simulink model "waveformSimulink_blocchi"  (R2019b)
settings: Solver=VariableStepAuto  StartTime=0.0  StopTime=1  RelTol=1e-3
values from neighbouring files (symbols this model uses):
  SNR = i    [start.m]
undefined symbols (not defined in the file or in its folder): Limit
libraries: commchan3 x4, commdigbbndcpm2 x4, dspsigops x4, commrandsrc3 x4, commsink2 x4, serdesDatapath x1
settings Model: Creator=boing  LastModifiedBy=Mattia

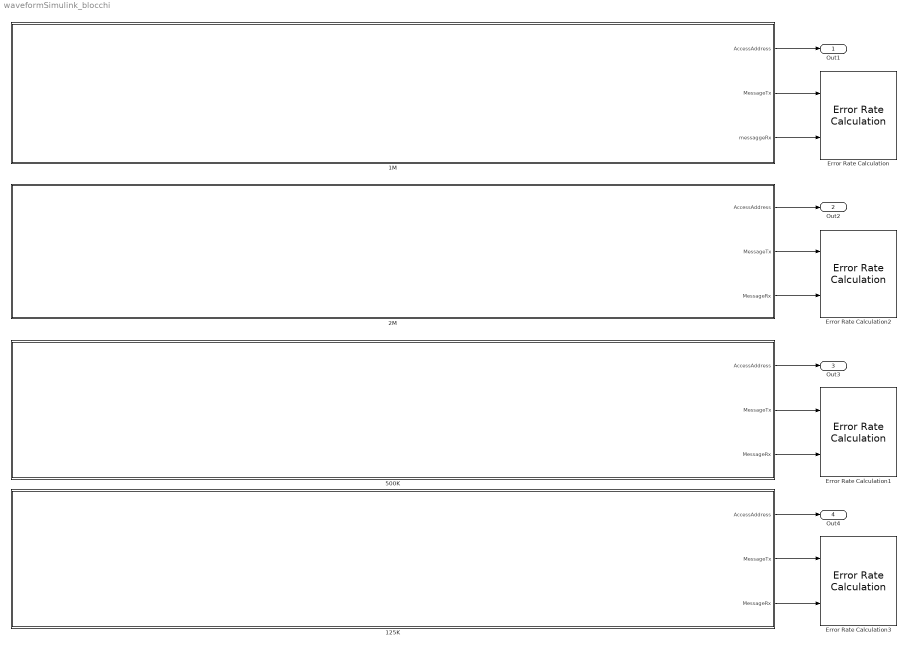
== system waveformSimulink_blocchi ==
  125K : Subsystem
  1M : Subsystem
  "2M " : Subsystem
  500K : Subsystem
  Error Rate Calculation : commsink2/Error Rate Calculation  N=0  st_delay=0  cp_mode=Entire frame  subframe=[]  PMode=Workspace  WsName=ErrorVec1M  RsMode2=off  stop=off  numErr=100  maxBits=1e6
      settings: SourceProductName=Communications Toolbox
  Error Rate Calculation1 : commsink2/Error Rate Calculation  N=0  st_delay=0  cp_mode=Entire frame  subframe=[]  PMode=Workspace  WsName=ErrorVec500K  RsMode2=off  stop=off  numErr=100  maxBits=1e6
      settings: SourceProductName=Communications Toolbox
  Error Rate Calculation2 : commsink2/Error Rate Calculation  N=0  st_delay=0  cp_mode=Entire frame  subframe=[]  PMode=Workspace  WsName=ErrorVec2M  RsMode2=off  stop=off  numErr=100  maxBits=1e6
      settings: SourceProductName=Communications Toolbox
  Error Rate Calculation3 : commsink2/Error Rate Calculation  N=0  st_delay=0  cp_mode=Entire frame  subframe=[]  PMode=Workspace  WsName=ErrorVec125K  RsMode2=off  stop=off  numErr=100  maxBits=1e6
      settings: SourceProductName=Communications Toolbox
  Out1 : Outport
  Out2 : Outport  Port=2
  Out3 : Outport  Port=3
  Out4 : Outport  Port=4
  wires:
  1M/2("MessageTx ") -> Error Rate Calculation/1
  1M/3(messaggeRx) -> Error Rate Calculation/2
  1M/1(AccessAddress) -> Out1/1
  500K/2(MessageTx) -> Error Rate Calculation1/1
  500K/3(MessageRx) -> Error Rate Calculation1/2
  "2M "/1(AccessAddress) -> Out2/1
  500K/1(AccessAddress) -> Out3/1
  "2M "/3(MessageRx) -> Error Rate Calculation2/2
  "2M "/2(MessageTx) -> Error Rate Calculation2/1
  125K/2(MessageTx) -> Error Rate Calculation3/1
  125K/3(MessageRx) -> Error Rate Calculation3/2
  125K/1(AccessAddress) -> Out4/1

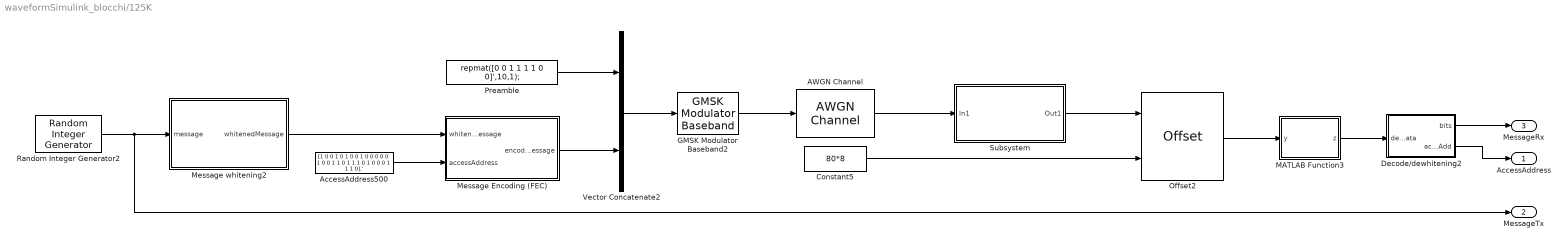
== system waveformSimulink_blocchi/125K ==
  AWGN Channel : commchan3/AWGN Channel  InputProcessing=Columns as channels (frame based)  seed=67  noiseMode="Signal to noise ratio  (SNR)"  EbNodB=10  EsNodB=10  SNRdB=SNR - 3  bitsPerSym=1  Ps=1  Tsym=1  variance=1
      settings: SourceProductName=Communications Toolbox
  AccessAddress500 : Constant  Value=[1 0 0 1 0 1 0 0 1 0 0 0 0 0 1 0 0 1 1 0 1 1 1 0 1 0 0 0 1 1 1 0].'  VectorParams1D=off
  Constant5 : Constant  Value=80*8
  Decode/dewhitening2 : MATLAB Function  TreatAsAtomicUnit=on
  GMSK Modulator Baseband2 : commdigbbndcpm2/GMSK Modulator Baseband  inputType=Bit  BT=0.5  pulseLength=1  preHistory=1  phaseOffset=4  samplesPerSymbol=8  RateOptions=Enforce single-rate processing  outDataType=double
      settings: SourceProductName=Communications Toolbox  SourceProductBaseCode=CM
  MATLAB Function3 : MATLAB Function  TreatAsAtomicUnit=on
  Message Encoding (FEC) : MATLAB Function  TreatAsAtomicUnit=on
  Message whitening2 : MATLAB Function  TreatAsAtomicUnit=on
  Offset2 : dspsigops/Offset  mode=Remove beginning samples  numDatOffPair=1  outWidthSpec=User-defined  outWidth=66560  actionOutRange=Clip
      settings: SourceProductName=DSP System Toolbox  SourceProductBaseCode=DS
  Preamble : Constant  Value=repmat([0 0 1 1 1 1 0 0]',10,1);
  Random Integer Generator2 : commrandsrc3/Random Integer Generator  SetSize=2  SeedSource=Auto  Seed=0  SampleTime=8*(10^-6)  SamplesPerFrame=1000  OutputDataType=double  SimulateUsing=Interpreted execution
      settings: SourceProductName=Communications Toolbox
  Subsystem : Subsystem
  Vector Concatenate2 : Concatenate
  AccessAddress : Outport
  MessageTx : Outport  Port=2
  MessageRx : Outport  Port=3
  wires:
  Vector Concatenate2/1 -> GMSK Modulator Baseband2/1
  Constant5/1 -> Offset2/2
  MATLAB Function3/1(z) -> Decode/dewhitening2/1(demodData)
  Decode/dewhitening2/1(bits) -> MessageRx/1
  Random Integer Generator2/1 -> MessageTx/1, Message whitening2/1(message)
  Offset2/1 -> MATLAB Function3/1(y)
  AccessAddress500/1 -> Message Encoding (FEC)/2(accessAddress)
  Decode/dewhitening2/2(accessAdd) -> AccessAddress/1
  Message Encoding (FEC)/1(encodedMessage) -> Vector Concatenate2/2
  Message whitening2/1(whitenedMessage) -> Message Encoding (FEC)/1(whitenedMessage)
  Preamble/1 -> Vector Concatenate2/1
  GMSK Modulator Baseband2/1 -> AWGN Channel/1
  AWGN Channel/1 -> Subsystem/1(In1)
  Subsystem/1(Out1) -> Offset2/1

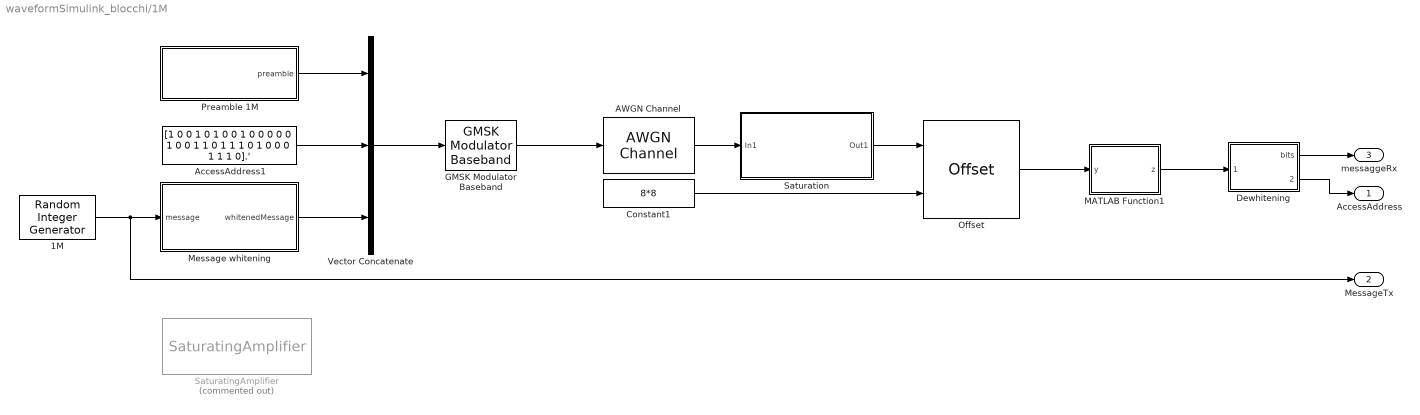
== system waveformSimulink_blocchi/1M ==
  1M : commrandsrc3/Random Integer Generator  SetSize=2  SeedSource=Auto  Seed=432234635  SampleTime=10^-6  SamplesPerFrame=1000  OutputDataType=double  SimulateUsing=Interpreted execution
      settings: SourceProductName=Communications Toolbox
  AWGN Channel : commchan3/AWGN Channel  InputProcessing=Columns as channels (frame based)  seed=67  noiseMode="Signal to noise ratio  (SNR)"  EbNodB=10  EsNodB=10  SNRdB=SNR  bitsPerSym=1  Ps=1  Tsym=1  variance=1
      settings: SourceProductName=Communications Toolbox
  "AccessAddress1 " : Constant  Value=[1 0 0 1 0 1 0 0 1 0 0 0 0 0 1 0 0 1 1 0 1 1 1 0 1 0 0 0 1 1 1 0].'  VectorParams1D=off
  Constant1 : Constant  Value=8*8
  Dewhitening : MATLAB Function  TreatAsAtomicUnit=on
  GMSK Modulator Baseband : commdigbbndcpm2/GMSK Modulator Baseband  inputType=Bit  BT=0.5  pulseLength=1  preHistory=1  phaseOffset=4  samplesPerSymbol=8  RateOptions=Enforce single-rate processing  outDataType=double
      settings: SourceProductName=Communications Toolbox  SourceProductBaseCode=CM
  MATLAB Function1 : MATLAB Function  TreatAsAtomicUnit=on
  Message whitening : MATLAB Function  TreatAsAtomicUnit=on
  Offset : dspsigops/Offset  mode=Remove beginning samples  numDatOffPair=1  outWidthSpec=User-defined  outWidth=8256  actionOutRange=Clip
      settings: SourceProductName=DSP System Toolbox  SourceProductBaseCode=DS
  Preamble 1M : MATLAB Function  TreatAsAtomicUnit=on
  SaturatingAmplifier : serdesDatapath/SaturatingAmplifier  Commented=on  InstantiateOnLoad=on  Mode=On  Specification=Limit and Linear Gain  Limit=1.2  LinearGain=1  VinVout=[ -2.4, -1.2; -1.92, -1.2; -1.44, -1.1328; -0.96, -0.86898; -0.48, -0.46862; 0, 0; 0.48, 0.46862; 0.96, 0.86898; 1.44, 1.1328; 1.92, 1.2; 2.4, 1.2 ]  ModeAMI=on  SavedName=SaturatingAmplifier
      settings: SourceProductName=SerDes Toolbox  SourceProductBaseCode=SX
  Saturation : Subsystem
  Vector Concatenate : Concatenate  NumInputs=3
  AccessAddress : Outport
  "MessageTx " : Outport  Port=2
  messaggeRx : Outport  Port=3
  wires:
  MATLAB Function1/1(z) -> Dewhitening/1(demodData)
  Message whitening/1(whitenedMessage) -> Vector Concatenate/3
  Offset/1 -> MATLAB Function1/1(y)
  Preamble 1M/1(preamble) -> Vector Concatenate/1
  Dewhitening/2(accessAdd) -> AccessAddress/1
  "AccessAddress1 "/1 -> Vector Concatenate/2
  Dewhitening/1(bits) -> messaggeRx/1
  Constant1/1 -> Offset/2
  Vector Concatenate/1 -> GMSK Modulator Baseband/1
  1M/1 -> "MessageTx "/1, Message whitening/1(message)
  GMSK Modulator Baseband/1 -> AWGN Channel/1
  AWGN Channel/1 -> Saturation/1(In1)
  Saturation/1(Out1) -> Offset/1

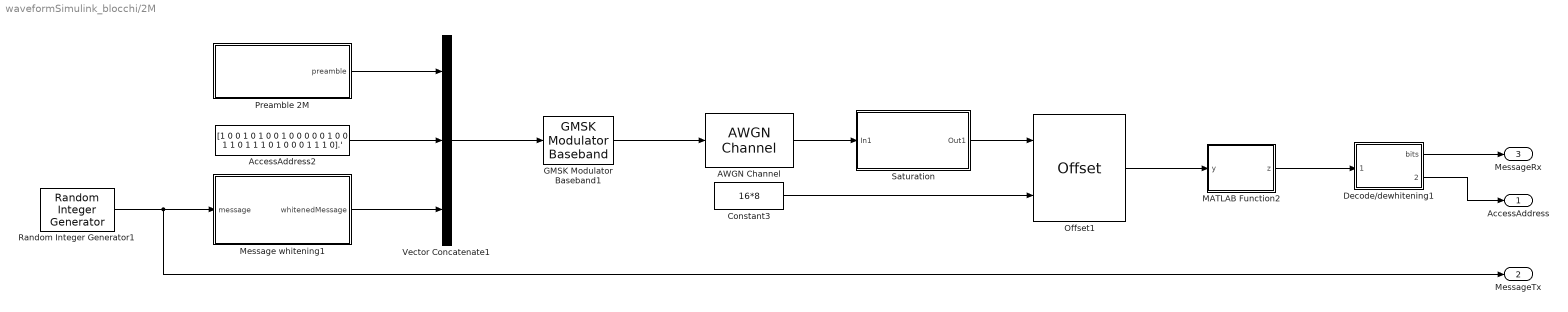
== system waveformSimulink_blocchi/2M  ==
  AWGN Channel : commchan3/AWGN Channel  InputProcessing=Columns as channels (frame based)  seed=67  noiseMode="Signal to noise ratio  (SNR)"  EbNodB=10  EsNodB=10  SNRdB=SNR  bitsPerSym=1  Ps=1  Tsym=1  variance=1
      settings: SourceProductName=Communications Toolbox
  AccessAddress2 : Constant  Value=[1 0 0 1 0 1 0 0 1 0 0 0 0 0 1 0 0 1 1 0 1 1 1 0 1 0 0 0 1 1 1 0].'  VectorParams1D=off
  Constant3 : Constant  Value=16*8
  Decode/dewhitening1 : MATLAB Function  TreatAsAtomicUnit=on
  GMSK Modulator Baseband1 : commdigbbndcpm2/GMSK Modulator Baseband  inputType=Bit  BT=0.5  pulseLength=1  preHistory=1  phaseOffset=4  samplesPerSymbol=8  RateOptions=Enforce single-rate processing  outDataType=double
      settings: SourceProductName=Communications Toolbox  SourceProductBaseCode=CM
  MATLAB Function2 : MATLAB Function  TreatAsAtomicUnit=on
  Message whitening1 : MATLAB Function  TreatAsAtomicUnit=on
  Offset1 : dspsigops/Offset  mode=Remove beginning samples  numDatOffPair=1  outWidthSpec=User-defined  outWidth=8256  actionOutRange=Clip
      settings: SourceProductName=DSP System Toolbox  SourceProductBaseCode=DS
  Preamble 2M : MATLAB Function  TreatAsAtomicUnit=on
  Random Integer Generator1 : commrandsrc3/Random Integer Generator  SetSize=2  SeedSource=Auto  Seed=0  SampleTime=0.5*(10^-6)  SamplesPerFrame=1000  OutputDataType=double  SimulateUsing=Interpreted execution
      settings: SourceProductName=Communications Toolbox
  "Saturation " : Subsystem
  Vector Concatenate1 : Concatenate  NumInputs=3
  AccessAddress : Outport
  MessageTx : Outport  Port=2
  MessageRx : Outport  Port=3
  wires:
  AccessAddress2/1 -> Vector Concatenate1/2
  Constant3/1 -> Offset1/2
  Preamble 2M/1(preamble) -> Vector Concatenate1/1
  Decode/dewhitening1/1(bits) -> MessageRx/1
  MATLAB Function2/1(z) -> Decode/dewhitening1/1(demodData)
  Vector Concatenate1/1 -> GMSK Modulator Baseband1/1
  Random Integer Generator1/1 -> MessageTx/1, Message whitening1/1(message)
  Decode/dewhitening1/2(accessAdd) -> AccessAddress/1
  Offset1/1 -> MATLAB Function2/1(y)
  Message whitening1/1(whitenedMessage) -> Vector Concatenate1/3
  GMSK Modulator Baseband1/1 -> AWGN Channel/1
  AWGN Channel/1 -> "Saturation "/1(In1)
  "Saturation "/1(Out1) -> Offset1/1

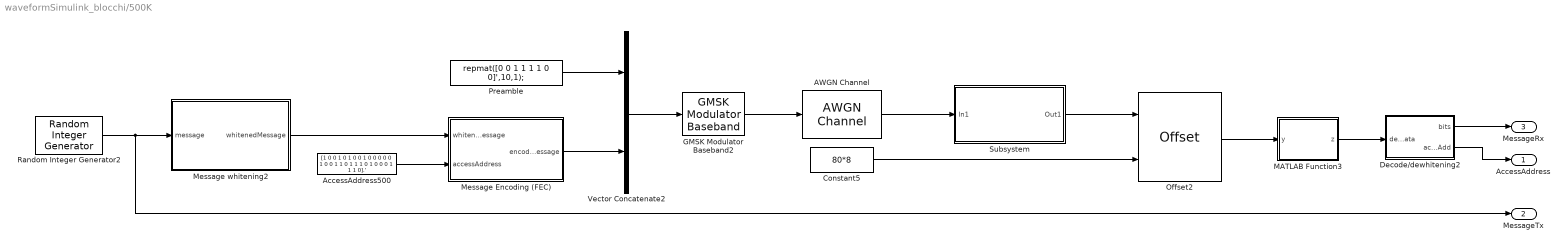
== system waveformSimulink_blocchi/500K ==
  AWGN Channel : commchan3/AWGN Channel  InputProcessing=Columns as channels (frame based)  seed=67  noiseMode="Signal to noise ratio  (SNR)"  EbNodB=10  EsNodB=10  SNRdB=SNR - 3  bitsPerSym=1  Ps=1  Tsym=1  variance=1
      settings: SourceProductName=Communications Toolbox
  AccessAddress500 : Constant  Value=[1 0 0 1 0 1 0 0 1 0 0 0 0 0 1 0 0 1 1 0 1 1 1 0 1 0 0 0 1 1 1 0].'  VectorParams1D=off
  Constant5 : Constant  Value=80*8
  Decode/dewhitening2 : MATLAB Function  TreatAsAtomicUnit=on
  GMSK Modulator Baseband2 : commdigbbndcpm2/GMSK Modulator Baseband  inputType=Bit  BT=0.5  pulseLength=1  preHistory=1  phaseOffset=4  samplesPerSymbol=8  RateOptions=Enforce single-rate processing  outDataType=double
      settings: SourceProductName=Communications Toolbox  SourceProductBaseCode=CM
  MATLAB Function3 : MATLAB Function  TreatAsAtomicUnit=on
  Message Encoding (FEC) : MATLAB Function  TreatAsAtomicUnit=on
  Message whitening2 : MATLAB Function  TreatAsAtomicUnit=on
  Offset2 : dspsigops/Offset  mode=Remove beginning samples  numDatOffPair=1  outWidthSpec=User-defined  outWidth=18416  actionOutRange=Clip
      settings: SourceProductName=DSP System Toolbox  SourceProductBaseCode=DS
  Preamble : Constant  Value=repmat([0 0 1 1 1 1 0 0]',10,1);
  Random Integer Generator2 : commrandsrc3/Random Integer Generator  SetSize=2  SeedSource=Auto  Seed=0  SampleTime=2*(10^-6)  SamplesPerFrame=1000  OutputDataType=double  SimulateUsing=Interpreted execution
      settings: SourceProductName=Communications Toolbox
  Subsystem : Subsystem
  Vector Concatenate2 : Concatenate
  AccessAddress : Outport
  MessageTx : Outport  Port=2
  MessageRx : Outport  Port=3
  wires:
  Vector Concatenate2/1 -> GMSK Modulator Baseband2/1
  Constant5/1 -> Offset2/2
  MATLAB Function3/1(z) -> Decode/dewhitening2/1(demodData)
  Decode/dewhitening2/1(bits) -> MessageRx/1
  Random Integer Generator2/1 -> MessageTx/1, Message whitening2/1(message)
  Offset2/1 -> MATLAB Function3/1(y)
  AccessAddress500/1 -> Message Encoding (FEC)/2(accessAddress)
  Decode/dewhitening2/2(accessAdd) -> AccessAddress/1
  Message Encoding (FEC)/1(encodedMessage) -> Vector Concatenate2/2
  Message whitening2/1(whitenedMessage) -> Message Encoding (FEC)/1(whitenedMessage)
  Preamble/1 -> Vector Concatenate2/1
  GMSK Modulator Baseband2/1 -> AWGN Channel/1
  AWGN Channel/1 -> Subsystem/1(In1)
  Subsystem/1(Out1) -> Offset2/1

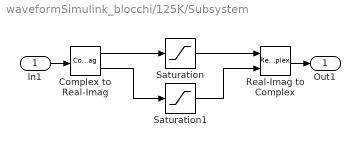
== system waveformSimulink_blocchi/125K/Subsystem ==
  In1 : Inport
  Complex to Real-Imag : ComplexToRealImag
  Real-Imag to Complex : RealImagToComplex
  Saturation : Saturate  UpperLimit=Limit  LowerLimit=-Limit
  Saturation1 : Saturate  UpperLimit=Limit  LowerLimit=-Limit
  Out1 : Outport
  wires:
  Complex to Real-Imag/1 -> Saturation/1
  Real-Imag to Complex/1 -> Out1/1
  Saturation/1 -> Real-Imag to Complex/1
  Saturation1/1 -> Real-Imag to Complex/2
  In1/1 -> Complex to Real-Imag/1
  Complex to Real-Imag/2 -> Saturation1/1

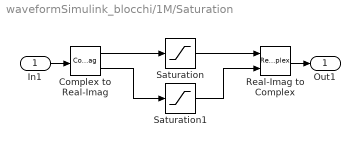
== system waveformSimulink_blocchi/1M/Saturation ==
  In1 : Inport
  Complex to Real-Imag : ComplexToRealImag
  Real-Imag to Complex : RealImagToComplex
  Saturation : Saturate  UpperLimit=Limit  LowerLimit=-Limit
  Saturation1 : Saturate  UpperLimit=Limit  LowerLimit=-Limit
  Out1 : Outport
  wires:
  Complex to Real-Imag/1 -> Saturation/1
  Real-Imag to Complex/1 -> Out1/1
  Saturation1/1 -> Real-Imag to Complex/2
  In1/1 -> Complex to Real-Imag/1
  Complex to Real-Imag/2 -> Saturation1/1
  Saturation/1 -> Real-Imag to Complex/1

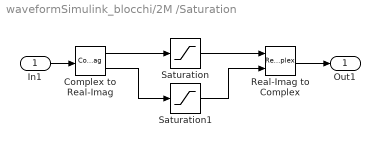
== system waveformSimulink_blocchi/2M /Saturation  ==
  In1 : Inport
  Complex to Real-Imag : ComplexToRealImag
  Real-Imag to Complex : RealImagToComplex
  Saturation : Saturate  UpperLimit=Limit  LowerLimit=-Limit
  Saturation1 : Saturate  UpperLimit=Limit  LowerLimit=-Limit
  Out1 : Outport
  wires:
  In1/1 -> Complex to Real-Imag/1
  Complex to Real-Imag/2 -> Saturation1/1
  Complex to Real-Imag/1 -> Saturation/1
  Saturation1/1 -> Real-Imag to Complex/2
  Real-Imag to Complex/1 -> Out1/1
  Saturation/1 -> Real-Imag to Complex/1

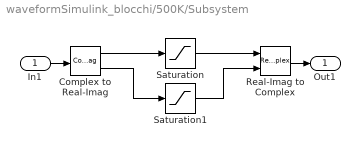
== system waveformSimulink_blocchi/500K/Subsystem ==
  In1 : Inport
  Complex to Real-Imag : ComplexToRealImag
  Real-Imag to Complex : RealImagToComplex
  Saturation : Saturate  UpperLimit=Limit  LowerLimit=-Limit
  Saturation1 : Saturate  UpperLimit=Limit  LowerLimit=-Limit
  Out1 : Outport
  wires:
  Complex to Real-Imag/2 -> Saturation1/1
  Complex to Real-Imag/1 -> Saturation/1
  Saturation1/1 -> Real-Imag to Complex/2
  Saturation/1 -> Real-Imag to Complex/1
  Real-Imag to Complex/1 -> Out1/1
  In1/1 -> Complex to Real-Imag/1

== matlab function waveformSimulink_blocchi/1M/Dewhitening ==
  data: demodData input; bits output double; accessAdd output
function [bits, accessAdd] = fcn(demodData)

accessAddLen = 32;      % Access address length in bits
chanIdx = 37;

% Demodulate and decodeaccessAdd
% if any(strcmp(phyMode,{'LE1M','LE2M'}))         % For LE1M or LE2M
accessAdd = int8(demodData(1:accessAddLen)>0);
decodeData = int8(demodData(1+accessAddLen:end)>0);
% else                                            % For LE500K or LE125K
%     [decodeData,accessAdd] = ble.internal.decode(demodData,phyMode);
% end

% Perform data dewhitening
dewhitenStateLen = 6;
chanIdxBin = comm.internal.utilities.de2biBase2LeftMSB(chanIdx,dewhitenStateLen);
initState = [1 chanIdxBin]; % Initial conditions of shift register
bits = double(ble.internal.whiten(decodeData,initState));

== matlab function waveformSimulink_blocchi/1M/Preamble 1M ==
  data: preamble output
function preamble = preamble
phyMode = "LE1M";
accessAddress = [1 0 0 1 0 1 0 0 1 0 0 0 0 0 1 0 0 1 1 0 1 1 1 0 1 0 0 0 1 1 1 0].';
preamble = ble.internal.preambleGenerator(phyMode,accessAddress);

== matlab function waveformSimulink_blocchi/2M /Message whitening1 ==
  data: message input; whitenedMessage output
function whitenedMessage = fcn(message)

chanIndCastToDouble = double(37);
chanIdxBin = comm.internal.utilities.de2biBase2LeftMSB(chanIndCastToDouble,6);
initState = [1 chanIdxBin];     % Initial conditions of shift register
whitenedMessage = ble.internal.whiten(message,initState);

== matlab function waveformSimulink_blocchi/1M/Message whitening ==
  data: message input; whitenedMessage output
function whitenedMessage = fcn(message)

chanIndCastToDouble = double(37);
chanIdxBin = comm.internal.utilities.de2biBase2LeftMSB(chanIndCastToDouble,6);
initState = [1 chanIdxBin];     % Initial conditions of shift register
whitenedMessage = ble.internal.whiten(message,initState);

== matlab function waveformSimulink_blocchi/1M/MATLAB Function1 ==
  data: y input; z output
function z = gmskdemod(y)
%GMSKDEMOD Gaussian minimum shift keying demodulation
%
%   Note: This is an internal undocumented function and its API and/or
%   functionality may change in subsequent releases.
%
%   Z = gmskdemod(Y,NSAMP) demodulates the complex envelope Y of a signal
%   using the Gaussian minimum shift keying method and produces soft
%   output Z. NSAMP denotes the number of samples per symbol and must be a
%   positive integer.

%   Copyright 2018 The MathWorks, Inc.

%#codegen
nSamp = 8;
sigLen = size(y,1);   % signal length in samples
nBits = sigLen/nSamp;  % signal length in bits

% Prepend the state
ini_state = complex(zeros(nSamp,1));
y = [ini_state;y];

% Perform gaussian matched filtering
bt = 0.5;
filtLen = 2*nSamp+1;
t = linspace(-1,1,filtLen);
alpha = sqrt(log(2)/2)/(bt);
h = (sqrt(pi)/alpha)*exp(-(t*pi/alpha).^2);
hNorm = h./sum(h);
yConv = conv2(y,hNorm(:),'same');

% Multiply the received GMSK signal by cos(pi*t/2T) and sin(pi*t/2T), where
% T is the symbol time. The phase offsets are different for the cos and
% sin multipliers to account for the circular shift in the I channel.
% These cos() and sin() multipliers are matched to the I and Q pulse
% shapes, respectively. Then perform receiver filtering. Assume that the
% received signal already is properly synchronized.

arg = pi * (0 : sigLen+nSamp-1)' / (2*nSamp);
multSig = complex(cos(arg+pi/2) .* real(yConv), sin(arg-pi/2) .* imag(yConv));

% Perform ideal integration
filtSig = (cumsum(multSig,1) - cumsum([zeros(2*nSamp,1); ...
    multSig(1:end-2*nSamp,:)],1)) / nSamp;

% Make I start from 2*nSamp and Q start from 3*nSamp. Account for the fact
% that the signal vector has been augmented in length.
Istart = 2 * nSamp;
Qstart = 3 * nSamp;
if (2*round(nBits/2) == nBits)
    Iend = sigLen;
    Qend = sigLen + nSamp;
else
    Iend = sigLen + nSamp;
    Qend = sigLen;
end

% Soft GMSK demodulation
zRealDec = real(filtSig(Istart:2*nSamp:Iend,:));
zImagDec = imag(filtSig(Qstart:2*nSamp:Qend,:));

% Upsample (i.e. repeat) the I and Q channels by 2, and shift the Q channel
% by 1 sample relative to the I channel. This operation allows for 2-bit
% decisions to be made over each I or Q symbol. Also, set the threshold
% for a suboptimal decision on the last bit.
zRealDec = kron(zRealDec,ones(2, 1));
zImagDec = kron(zImagDec,ones(2, 1));

if 2*round(nBits/2) == nBits
    threshold = 0.5 * sum(double(sign(real(filtSig(end-nSamp+1:end,:)))))/nSamp;
    zRealDec = [zRealDec(2:end,:); ...
        double(sign( real(filtSig(end,:)) - threshold ))];
else
    zRealDec = zRealDec(2:end,:);
    threshold = 0.5 * sum(double(sign(imag(filtSig(end-nSamp+1:end,:)))))/nSamp;
    zImagDec = [zImagDec; ...
    double(sign( imag(filtSig(end,:)) - threshold ))];
end

% Now multiply the real and imaginary parts together to find the signed
% data values
z = -zRealDec .* zImagDec;

end

== matlab function waveformSimulink_blocchi/2M /Preamble 2M ==
  data: preamble output
function preamble = preamble
phyMode = "LE2M";
accessAddress = [1 0 0 1 0 1 0 0 1 0 0 0 0 0 1 0 0 1 1 0 1 1 1 0 1 0 0 0 1 1 1 0].';
preamble = ble.internal.preambleGenerator(phyMode,accessAddress);

== matlab function waveformSimulink_blocchi/2M /Decode//dewhitening1 ==
  data: demodData input; bits output double; accessAdd output
function [bits, accessAdd] = fcn(demodData)

accessAddLen = 32;      % Access address length in bits
chanIdx = 37;

% Demodulate and decodeaccessAdd
% if any(strcmp(phyMode,{'LE1M','LE2M'}))         % For LE1M or LE2M
accessAdd = int8(demodData(1:accessAddLen)>0);
decodeData = int8(demodData(1+accessAddLen:end)>0);
% else                                            % For LE500K or LE125K
%     [decodeData,accessAdd] = ble.internal.decode(demodData,phyMode);
% end

% Perform data dewhitening
dewhitenStateLen = 6;
chanIdxBin = comm.internal.utilities.de2biBase2LeftMSB(chanIdx,dewhitenStateLen);
initState = [1 chanIdxBin]; % Initial conditions of shift register
bits = double(ble.internal.whiten(decodeData,initState));

== matlab function waveformSimulink_blocchi/2M /MATLAB Function2 ==
  data: y input; z output
function z = gmskdemod(y)
%GMSKDEMOD Gaussian minimum shift keying demodulation
%
%   Note: This is an internal undocumented function and its API and/or
%   functionality may change in subsequent releases.
%
%   Z = gmskdemod(Y,NSAMP) demodulates the complex envelope Y of a signal
%   using the Gaussian minimum shift keying method and produces soft
%   output Z. NSAMP denotes the number of samples per symbol and must be a
%   positive integer.

%   Copyright 2018 The MathWorks, Inc.

%#codegen
nSamp = 8;
sigLen = size(y,1);   % signal length in samples
nBits = sigLen/nSamp;  % signal length in bits

% Prepend the state
ini_state = complex(zeros(nSamp,1));
y = [ini_state;y];

% Perform gaussian matched filtering
bt = 0.5;
filtLen = 2*nSamp+1;
t = linspace(-1,1,filtLen);
alpha = sqrt(log(2)/2)/(bt);
h = (sqrt(pi)/alpha)*exp(-(t*pi/alpha).^2);
hNorm = h./sum(h);
yConv = conv2(y,hNorm(:),'same');

% Multiply the received GMSK signal by cos(pi*t/2T) and sin(pi*t/2T), where
% T is the symbol time. The phase offsets are different for the cos and
% sin multipliers to account for the circular shift in the I channel.
% These cos() and sin() multipliers are matched to the I and Q pulse
% shapes, respectively. Then perform receiver filtering. Assume that the
% received signal already is properly synchronized.

arg = pi * (0 : sigLen+nSamp-1)' / (2*nSamp);
multSig = complex(cos(arg+pi/2) .* real(yConv), sin(arg-pi/2) .* imag(yConv));

% Perform ideal integration
filtSig = (cumsum(multSig,1) - cumsum([zeros(2*nSamp,1); ...
    multSig(1:end-2*nSamp,:)],1)) / nSamp;

% Make I start from 2*nSamp and Q start from 3*nSamp. Account for the fact
% that the signal vector has been augmented in length.
Istart = 2 * nSamp;
Qstart = 3 * nSamp;
if (2*round(nBits/2) == nBits)
    Iend = sigLen;
    Qend = sigLen + nSamp;
else
    Iend = sigLen + nSamp;
    Qend = sigLen;
end

% Soft GMSK demodulation
zRealDec = real(filtSig(Istart:2*nSamp:Iend,:));
zImagDec = imag(filtSig(Qstart:2*nSamp:Qend,:));

% Upsample (i.e. repeat) the I and Q channels by 2, and shift the Q channel
% by 1 sample relative to the I channel. This operation allows for 2-bit
% decisions to be made over each I or Q symbol. Also, set the threshold
% for a suboptimal decision on the last bit.
zRealDec = kron(zRealDec,ones(2, 1));
zImagDec = kron(zImagDec,ones(2, 1));

if 2*round(nBits/2) == nBits
    threshold = 0.5 * sum(double(sign(real(filtSig(end-nSamp+1:end,:)))))/nSamp;
    zRealDec = [zRealDec(2:end,:); ...
        double(sign( real(filtSig(end,:)) - threshold ))];
else
    zRealDec = zRealDec(2:end,:);
    threshold = 0.5 * sum(double(sign(imag(filtSig(end-nSamp+1:end,:)))))/nSamp;
    zImagDec = [zImagDec; ...
    double(sign( imag(filtSig(end,:)) - threshold ))];
end

% Now multiply the real and imaginary parts together to find the signed
% data values
z = -zRealDec .* zImagDec;

end

== matlab function waveformSimulink_blocchi/500K/Decode//dewhitening2 ==
  data: demodData input; bits output double; accessAdd output
function [bits, accessAdd] = fcn(demodData)

phyMode = 'LE500K';
chanIdx = 37;

% Demodulate and decodeaccessAdd
% if any(strcmp(phyMode,{'LE1M','LE2M'}))         % For LE1M or LE2M
% accessAdd = int8(demodData(1:accessAddLen)>0);
% decodeData = int8(demodData(1+accessAddLen:end)>0);
% else                                            % For LE500K or LE125K
[decodeData,accessAdd] = ble.internal.decode(demodData,phyMode);
% end

% Perform data dewhitening
dewhitenStateLen = 6;
chanIdxBin = comm.internal.utilities.de2biBase2LeftMSB(chanIdx,dewhitenStateLen);
initState = [1 chanIdxBin]; % Initial conditions of shift register
bits = double(ble.internal.whiten(decodeData,initState));

== matlab function waveformSimulink_blocchi/500K/MATLAB Function3 ==
  data: y input; z output
function z = gmskdemod(y)
%GMSKDEMOD Gaussian minimum shift keying demodulation
%
%   Note: This is an internal undocumented function and its API and/or
%   functionality may change in subsequent releases.
%
%   Z = gmskdemod(Y,NSAMP) demodulates the complex envelope Y of a signal
%   using the Gaussian minimum shift keying method and produces soft
%   output Z. NSAMP denotes the number of samples per symbol and must be a
%   positive integer.

%   Copyright 2018 The MathWorks, Inc.

%#codegen
nSamp = 8;
sigLen = size(y,1);   % signal length in samples
nBits = sigLen/nSamp;  % signal length in bits

% Prepend the state
ini_state = complex(zeros(nSamp,1));
y = [ini_state;y];

% Perform gaussian matched filtering
bt = 0.5;
filtLen = 2*nSamp+1;
t = linspace(-1,1,filtLen);
alpha = sqrt(log(2)/2)/(bt);
h = (sqrt(pi)/alpha)*exp(-(t*pi/alpha).^2);
hNorm = h./sum(h);
yConv = conv2(y,hNorm(:),'same');

% Multiply the received GMSK signal by cos(pi*t/2T) and sin(pi*t/2T), where
% T is the symbol time. The phase offsets are different for the cos and
% sin multipliers to account for the circular shift in the I channel.
% These cos() and sin() multipliers are matched to the I and Q pulse
% shapes, respectively. Then perform receiver filtering. Assume that the
% received signal already is properly synchronized.

arg = pi * (0 : sigLen+nSamp-1)' / (2*nSamp);
multSig = complex(cos(arg+pi/2) .* real(yConv), sin(arg-pi/2) .* imag(yConv));

% Perform ideal integration
filtSig = (cumsum(multSig,1) - cumsum([zeros(2*nSamp,1); ...
    multSig(1:end-2*nSamp,:)],1)) / nSamp;

% Make I start from 2*nSamp and Q start from 3*nSamp. Account for the fact
% that the signal vector has been augmented in length.
Istart = 2 * nSamp;
Qstart = 3 * nSamp;
if (2*round(nBits/2) == nBits)
    Iend = sigLen;
    Qend = sigLen + nSamp;
else
    Iend = sigLen + nSamp;
    Qend = sigLen;
end

% Soft GMSK demodulation
zRealDec = real(filtSig(Istart:2*nSamp:Iend,:));
zImagDec = imag(filtSig(Qstart:2*nSamp:Qend,:));

% Upsample (i.e. repeat) the I and Q channels by 2, and shift the Q channel
% by 1 sample relative to the I channel. This operation allows for 2-bit
% decisions to be made over each I or Q symbol. Also, set the threshold
% for a suboptimal decision on the last bit.
zRealDec = kron(zRealDec,ones(2, 1));
zImagDec = kron(zImagDec,ones(2, 1));

if 2*round(nBits/2) == nBits
    threshold = 0.5 * sum(double(sign(real(filtSig(end-nSamp+1:end,:)))))/nSamp;
    zRealDec = [zRealDec(2:end,:); ...
        double(sign( real(filtSig(end,:)) - threshold ))];
else
    zRealDec = zRealDec(2:end,:);
    threshold = 0.5 * sum(double(sign(imag(filtSig(end-nSamp+1:end,:)))))/nSamp;
    zImagDec = [zImagDec; ...
    double(sign( imag(filtSig(end,:)) - threshold ))];
end

% Now multiply the real and imaginary parts together to find the signed
% data values
z = -zRealDec .* zImagDec;

end

== matlab function waveformSimulink_blocchi/500K/Message whitening2 ==
  data: message input; whitenedMessage output
function whitenedMessage = fcn(message)

chanIndCastToDouble = double(37);
chanIdxBin = comm.internal.utilities.de2biBase2LeftMSB(chanIndCastToDouble,6);
initState = [1 chanIdxBin];     % Initial conditions of shift register
whitenedMessage = ble.internal.whiten(message,initState);

== matlab function waveformSimulink_blocchi/500K/Message Encoding (FEC) ==
  data: whitenedMessage input; encodedMessage output; accessAddress input
function encodedMessage = fcn(whitenedMessage, accessAddress)

codingIndicator = [0 0]';
encodedMessage = double(ble.internal.encode(whitenedMessage,accessAddress,...
                            codingIndicator));

== matlab function waveformSimulink_blocchi/125K/Decode//dewhitening2 ==
  data: demodData input; bits output double; accessAdd output
function [bits, accessAdd] = fcn(demodData)

phyMode = 'LE125K';
chanIdx = 37;

% Demodulate and decodeaccessAdd
% if any(strcmp(phyMode,{'LE1M','LE2M'}))         % For LE1M or LE2M
% accessAdd = int8(demodData(1:accessAddLen)>0);
% decodeData = int8(demodData(1+accessAddLen:end)>0);
% else                                            % For LE500K or LE125K
[decodeData,accessAdd] = ble.internal.decode(demodData,phyMode);
% end

% Perform data dewhitening
dewhitenStateLen = 6;
chanIdxBin = comm.internal.utilities.de2biBase2LeftMSB(chanIdx,dewhitenStateLen);
initState = [1 chanIdxBin]; % Initial conditions of shift register
bits = double(ble.internal.whiten(decodeData,initState));

== matlab function waveformSimulink_blocchi/125K/MATLAB Function3 ==
  data: y input; z output
function z = gmskdemod(y)
%GMSKDEMOD Gaussian minimum shift keying demodulation
%
%   Note: This is an internal undocumented function and its API and/or
%   functionality may change in subsequent releases.
%
%   Z = gmskdemod(Y,NSAMP) demodulates the complex envelope Y of a signal
%   using the Gaussian minimum shift keying method and produces soft
%   output Z. NSAMP denotes the number of samples per symbol and must be a
%   positive integer.

%   Copyright 2018 The MathWorks, Inc.

%#codegen
nSamp = 8;
sigLen = size(y,1);   % signal length in samples
nBits = sigLen/nSamp;  % signal length in bits

% Prepend the state
ini_state = complex(zeros(nSamp,1));
y = [ini_state;y];

% Perform gaussian matched filtering
bt = 0.5;
filtLen = 2*nSamp+1;
t = linspace(-1,1,filtLen);
alpha = sqrt(log(2)/2)/(bt);
h = (sqrt(pi)/alpha)*exp(-(t*pi/alpha).^2);
hNorm = h./sum(h);
yConv = conv2(y,hNorm(:),'same');

% Multiply the received GMSK signal by cos(pi*t/2T) and sin(pi*t/2T), where
% T is the symbol time. The phase offsets are different for the cos and
% sin multipliers to account for the circular shift in the I channel.
% These cos() and sin() multipliers are matched to the I and Q pulse
% shapes, respectively. Then perform receiver filtering. Assume that the
% received signal already is properly synchronized.

arg = pi * (0 : sigLen+nSamp-1)' / (2*nSamp);
multSig = complex(cos(arg+pi/2) .* real(yConv), sin(arg-pi/2) .* imag(yConv));

% Perform ideal integration
filtSig = (cumsum(multSig,1) - cumsum([zeros(2*nSamp,1); ...
    multSig(1:end-2*nSamp,:)],1)) / nSamp;

% Make I start from 2*nSamp and Q start from 3*nSamp. Account for the fact
% that the signal vector has been augmented in length.
Istart = 2 * nSamp;
Qstart = 3 * nSamp;
if (2*round(nBits/2) == nBits)
    Iend = sigLen;
    Qend = sigLen + nSamp;
else
    Iend = sigLen + nSamp;
    Qend = sigLen;
end

% Soft GMSK demodulation
zRealDec = real(filtSig(Istart:2*nSamp:Iend,:));
zImagDec = imag(filtSig(Qstart:2*nSamp:Qend,:));

% Upsample (i.e. repeat) the I and Q channels by 2, and shift the Q channel
% by 1 sample relative to the I channel. This operation allows for 2-bit
% decisions to be made over each I or Q symbol. Also, set the threshold
% for a suboptimal decision on the last bit.
zRealDec = kron(zRealDec,ones(2, 1));
zImagDec = kron(zImagDec,ones(2, 1));

if 2*round(nBits/2) == nBits
    threshold = 0.5 * sum(double(sign(real(filtSig(end-nSamp+1:end,:)))))/nSamp;
    zRealDec = [zRealDec(2:end,:); ...
        double(sign( real(filtSig(end,:)) - threshold ))];
else
    zRealDec = zRealDec(2:end,:);
    threshold = 0.5 * sum(double(sign(imag(filtSig(end-nSamp+1:end,:)))))/nSamp;
    zImagDec = [zImagDec; ...
    double(sign( imag(filtSig(end,:)) - threshold ))];
end

% Now multiply the real and imaginary parts together to find the signed
% data values
z = -zRealDec .* zImagDec;

end

== matlab function waveformSimulink_blocchi/125K/Message Encoding (FEC) ==
  data: whitenedMessage input; encodedMessage output; accessAddress input
function encodedMessage = fcn(whitenedMessage, accessAddress)

codingIndicator = [0 1]';
encodedMessage = double(ble.internal.encode(whitenedMessage,accessAddress,...
                            codingIndicator));

== matlab function waveformSimulink_blocchi/125K/Message whitening2 ==
  data: message input; whitenedMessage output
function whitenedMessage = fcn(message)

chanIndCastToDouble = double(37);
chanIdxBin = comm.internal.utilities.de2biBase2LeftMSB(chanIndCastToDouble,6);
initState = [1 chanIdxBin];     % Initial conditions of shift register
whitenedMessage = ble.internal.whiten(message,initState);
